simulink model "flatearth_model"  (R2018a)
settings: Solver=VariableStepAuto  StartTime=0.0  StopTime=16.5  RelTol=1e-3
libraries: shared6dof x1, aerolibanim x1, simulink x1
settings Model: PauseTimes=2.5  Creator=annakooperberg  LastModifiedBy=annakooperberg

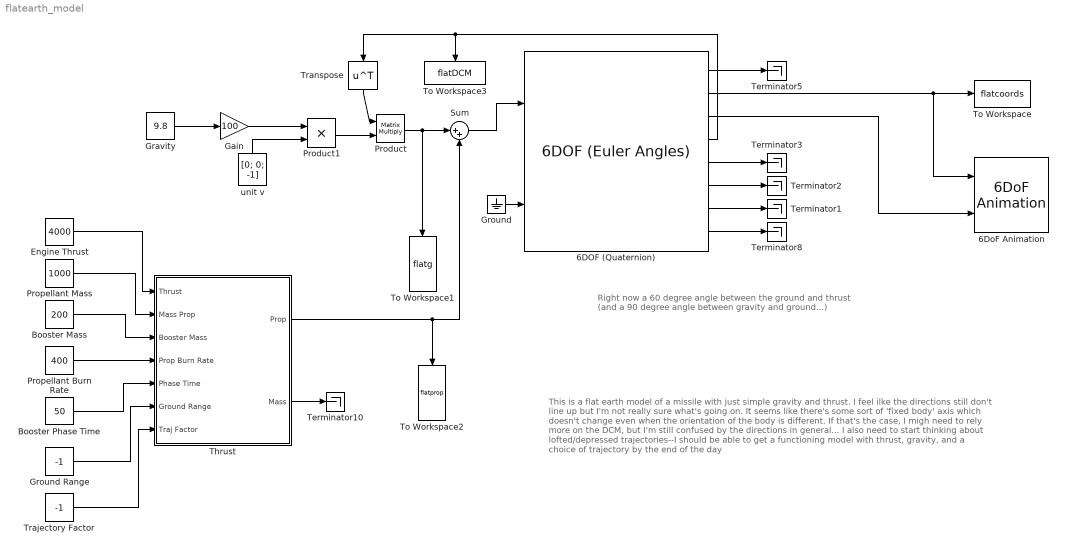
== system flatearth_model ==
  note: Right now a 60 degree angle between the ground and thrust
      | (and a 90 degree angle between gravity and ground...)
  note: This is a flat earth model of a missile with just simple gravity and thrust. I feel ilke the directions
      | still don't line up but I'm not really sure what's going on. It seems like there's some sort of 'fixed body'
      | axis which doesn't change even when the orientation of the body is different. If that's the case, I migh
      | need to rely more on the DCM, but I'm still confused by the directions in general... I also need to start thinking
      | about lofted/depressed trajectories--I should be able to get a functioning model with thrust, gravity, and a choice
      | of trajectory by the end of the day
  6DOF (Quaternion) : shared6dof/6DOF (Euler Angles)  units=Metric (MKS)  mtype=Fixed  rep=Quaternion  xme_0=[0 0 0]  Vm_0=[0 0 0]  eul_0=[0 pi/2 0]  pm_0=[0 0 0]  mass_0=100  mass_e=0.5  mass_f=2.0  inertia=eye(3)  inertia_e=eye(3)  inertia_f=2*eye(3)  k_quat=1.0  vre_flag=on  abi_flag=off  aMode=0
      settings: SourceProductBaseCode=AE
  6DoF Animation : aerolibanim/6DoF Animation  u1=[-2000 2000 -2000 2000 -2000 2000]  u2=0.1  u3=150  u4=[4000 0 -5000]  u5=Fixed position  u6=[2000 500 -3150]  u7=10  u8=on
      settings: SourceProductName=Aerospace Blockset
  Booster Mass : Constant  Value=200
  Booster Phase Time : Constant  Value=50
  Engine Thrust : Constant  Value=4000
  Gain : Gain  Gain=100
  Gravity : Constant  Value=9.8
  Ground : Ground
  Ground Range : Constant  Value=-1
  Product : Product  Multiplication=Matrix(*)
  Product1 : Product
  Propellant Burn Rate : Constant  Value=400
  Propellant Mass : Constant  Value=1000
  Sum : Sum  Inputs=|++
  Terminator{1..3,5,8,10} (6 alike) : Terminator
  Thrust : Subsystem
  To Workspace : ToWorkspace  VariableName=flatcoords  SaveFormat=Timeseries  SampleTime=-1
  To Workspace1 : ToWorkspace  VariableName=flatg  SaveFormat=Timeseries  SampleTime=-1
  To Workspace2 : ToWorkspace  VariableName=flatprop  SaveFormat=Timeseries  SampleTime=-1
  To Workspace3 : ToWorkspace  VariableName=flatDCM  SaveFormat=Timeseries  SampleTime=-1
  Trajectory Factor : Constant  Value=-1
  Transpose : Math  Operator=transpose  SaturateOnIntegerOverflow=on
  unit v : Constant  Value=[0; 0; -1]
  wires:
  6DOF (Quaternion)/2 -> To Workspace/1, 6DoF Animation/1
  6DOF (Quaternion)/3 -> 6DoF Animation/2
  Ground/1 -> 6DOF (Quaternion)/2
  6DOF (Quaternion)/8 -> Terminator8/1
  6DOF (Quaternion)/7 -> Terminator1/1
  6DOF (Quaternion)/6 -> Terminator2/1
  6DOF (Quaternion)/5 -> Terminator3/1
  6DOF (Quaternion)/1 -> Terminator5/1
  Propellant Burn Rate/1 -> Thrust/4(Prop Burn Rate)
  Booster Mass/1 -> Thrust/3(Booster Mass)
  Thrust/2(Mass) -> Terminator10/1
  Booster Phase Time/1 -> Thrust/5(Phase Time)
  Trajectory Factor/1 -> Thrust/7(Traj Factor)
  Engine Thrust/1 -> Thrust/1(Thrust)
  Ground Range/1 -> Thrust/6(Ground Range)
  Propellant Mass/1 -> Thrust/2(Mass Prop)
  Thrust/1(Prop) -> Sum/2, To Workspace2/1
  Sum/1 -> 6DOF (Quaternion)/1
  Gravity/1 -> Gain/1
  Gain/1 -> Product1/1
  Product1/1 -> Product/2
  unit v/1 -> Product1/2
  Product/1 -> Sum/1, To Workspace1/1
  6DOF (Quaternion)/4 -> Transpose/1, To Workspace3/1
  Transpose/1 -> Product/1

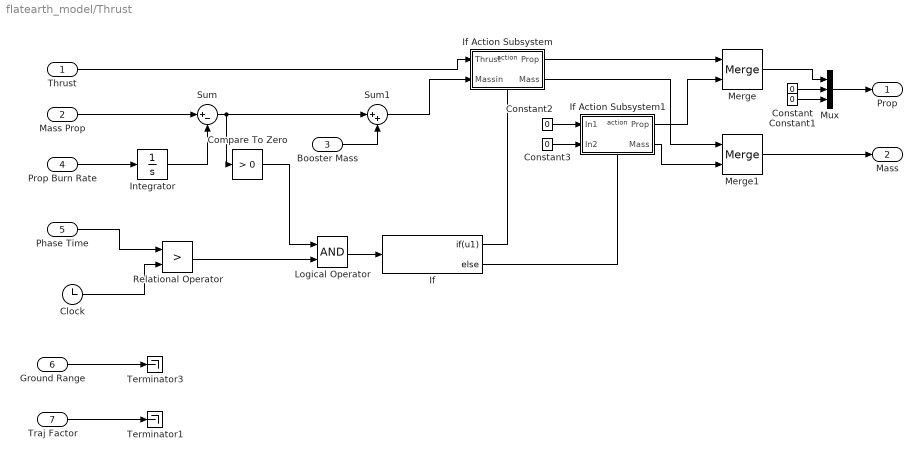
== system flatearth_model/Thrust ==
  Thrust : Inport
  Mass Prop : Inport  Port=2
  Booster Mass : Inport  Port=3
  Prop Burn Rate : Inport  Port=4
  Phase Time : Inport  Port=5
  Ground Range : Inport  Port=6
  Traj Factor : Inport  Port=7
  Clock : Clock
  Compare To Zero : simulink/Logic and Bit Operations/Compare To Zero  relop=>  OutDataTypeStr=boolean
  Constant{,1..3} (4 alike) : Constant  Value=0
  If : If  IfExpression=u1
  If Action Subsystem : Subsystem  TreatAsAtomicUnit=on
  If Action Subsystem1 : Subsystem  TreatAsAtomicUnit=on
  Integrator : Integrator
  Logical Operator : Logic  AllPortsSameDT=off  OutDataTypeStr=boolean
  Merge : Merge
  Merge1 : Merge
  Mux : Mux  Inputs=3
  Relational Operator : RelationalOperator  Operator=>  OutDataTypeStr=boolean  RndMeth=Nearest
  Sum : Sum  Inputs=|+-
  Sum1 : Sum  Inputs=|++
  Terminator1 : Terminator
  Terminator3 : Terminator
  Prop : Outport
  Mass : Outport  Port=2
  wires:
  Phase Time/1 -> Relational Operator/1
  If Action Subsystem/1(Prop) -> Merge/1
  Thrust/1 -> If Action Subsystem/1(Thrust)
  Mass Prop/1 -> Sum/1
  If/1 -> If Action Subsystem/Action
  Merge/1 -> Mux/1
  Compare To Zero/1 -> Logical Operator/1
  Clock/1 -> Relational Operator/2
  Relational Operator/1 -> Logical Operator/2
  Prop Burn Rate/1 -> Integrator/1
  If Action Subsystem1/1(Prop) -> Merge/2
  Constant1/1 -> Mux/3
  Mux/1 -> Prop/1
  If/2 -> If Action Subsystem1/Action
  Constant/1 -> Mux/2
  Sum/1 -> Sum1/1, Compare To Zero/1
  Logical Operator/1 -> If/1
  Integrator/1 -> Sum/2
  Sum1/1 -> If Action Subsystem/2(Massin)
  Booster Mass/1 -> Sum1/2
  If Action Subsystem/2(Mass) -> Merge1/1
  If Action Subsystem1/2(Mass) -> Merge1/2
  Merge1/1 -> Mass/1
  Constant3/1 -> If Action Subsystem1/2(In2)
  Constant2/1 -> If Action Subsystem1/1(In1)
  Traj Factor/1 -> Terminator1/1
  Ground Range/1 -> Terminator3/1

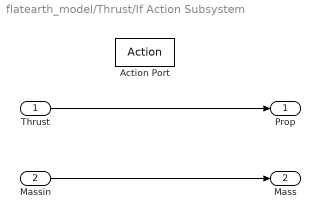
== system flatearth_model/Thrust/If Action Subsystem ==
  Thrust : Inport
  Massin : Inport  Port=2
  Action Port : ActionPort  ActionType=then
  Prop : Outport
  Mass : Outport  Port=2
  wires:
  Thrust/1 -> Prop/1
  Massin/1 -> Mass/1

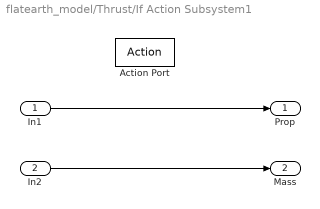
== system flatearth_model/Thrust/If Action Subsystem1 ==
  In1 : Inport
  In2 : Inport  Port=2
  Action Port : ActionPort  ActionType=else
  Prop : Outport
  Mass : Outport  Port=2
  wires:
  In1/1 -> Prop/1
  In2/1 -> Mass/1
